simulink model "pend"  (R2015a)
settings: Solver=ode45  StartTime=0.0  StopTime=2  RelTol=1e-3
values from neighbouring files (symbols this model uses):
  b = 0.1    [Pendulum.m]
  g = 9.8    [Pendulum.m]
  l = 0.5    [Pendulum.m]
  M = 0.5    [Pendulum.m]
  m = 0.4    [Pendulum.m]
settings Model: Creator=Simon  LastModifiedBy=Simon
settings DebuggingCC: InitInArrayFormatMsg=none

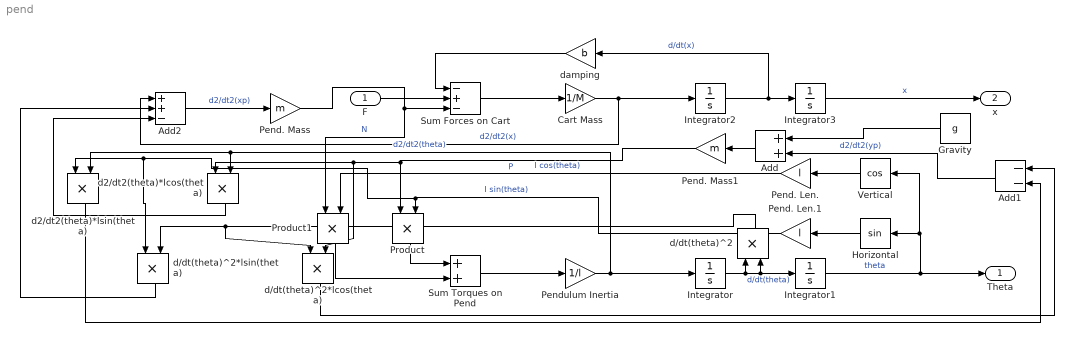
== system pend ==
  F : Inport
  Add : Sum
  Add1 : Sum  Inputs=--
  Add2 : Sum  Inputs=++-
  Cart Mass : Gain  Gain=1/M
  Gravity : Constant  Value=g
  Horizontal : Trigonometry
  Integrator{,1..3} (4 alike) : Integrator
  Pend. Len. : Gain  Gain=l
  Pend. Len.1 : Gain  Gain=l
  Pend. Mass : Gain  Gain=m
  Pend. Mass1 : Gain  Gain=m
  Pendulum Inertia : Gain  Gain=1/l
  Product : Product
  Product1 : Product
  Sum Forces on Cart : Sum  Inputs=-+-
  Sum Torques on Pend : Sum
  Vertical : Trigonometry  Operator=cos
  d/dt(theta)^2 : Product
  d/dt(theta)^2*lcos(theta) : Product
  d/dt(theta)^2*lsin(theta) : Product
  d2/dt2(theta)*lcos(theta) : Product
  d2/dt2(theta)*lsin(theta) : Product
  "damping " : Gain  Gain=b
  Theta : Outport
  x : Outport  Port=2
  wires:
  Integrator/1 -> d/dt(theta)^2/2, Integrator1/1, d/dt(theta)^2/1  "d/dt(theta)"
  Integrator1/1 -> Theta/1, Vertical/1, Horizontal/1  "theta"
  Pendulum Inertia/1 -> Integrator/1, d2/dt2(theta)*lcos(theta)/2, d2/dt2(theta)*lsin(theta)/2  "d2/dt2(theta)"
  Sum Torques on Pend/1 -> Pendulum Inertia/1
  Sum Forces on Cart/1 -> Cart Mass/1
  Integrator2/1 -> "damping "/1, Integrator3/1  "d/dt(x)"
  Cart Mass/1 -> Add2/1, Integrator2/1  "d2/dt2(x)"
  Integrator3/1 -> x/1  "x"
  "damping "/1 -> Sum Forces on Cart/1
  F/1 -> Sum Forces on Cart/2
  Vertical/1 -> Pend. Len./1
  Horizontal/1 -> Pend. Len.1/1
  Pend. Len./1 -> Product1/2  "I cos(theta)"
  Pend. Len.1/1 -> d/dt(theta)^2*lsin(theta)/1, d2/dt2(theta)*lsin(theta)/1, Product/2  "I sin(theta)"
  Product1/1 -> Sum Torques on Pend/2
  Product/1 -> Sum Torques on Pend/1
  Pend. Mass1/1 -> d2/dt2(theta)*lcos(theta)/1, d/dt(theta)^2*lcos(theta)/2, Product/1  "P"
  Pend. Mass/1 -> Product1/1, Sum Forces on Cart/3  "N"
  Add2/1 -> Pend. Mass/1  "d2/dt2(xp)"
  Add/1 -> Pend. Mass1/1
  Gravity/1 -> Add/1
  Add1/1 -> Add/2  "d2/dt2(yp)"
  d/dt(theta)^2/1 -> d/dt(theta)^2*lsin(theta)/2, d/dt(theta)^2*lcos(theta)/1
  d2/dt2(theta)*lsin(theta)/1 -> Add1/2
  d2/dt2(theta)*lcos(theta)/1 -> Add2/3
  d/dt(theta)^2*lcos(theta)/1 -> Add1/1
  d/dt(theta)^2*lsin(theta)/1 -> Add2/2
